simulink model "magnetorquer"  (R2021b)
settings: Solver=VariableStepAuto  StartTime=0.0  StopTime=10.0  RelTol=1e-3
libraries: matrix_library x2
settings Model: Creator=jorgemarrero  LastModifiedBy=jorgemarrero

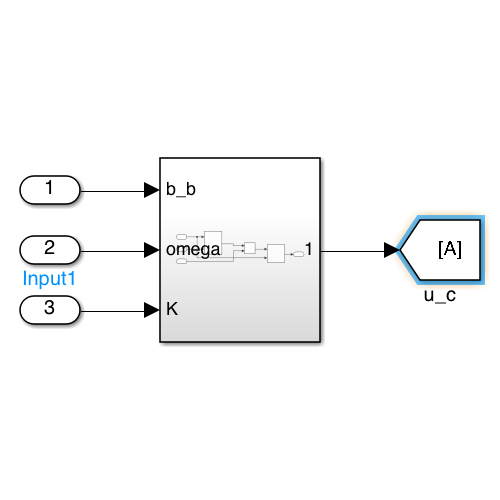
[thumbnail: Simulink's stored preview of the top-level diagram]
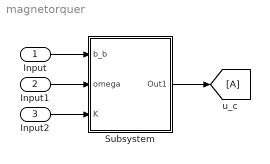
== system magnetorquer ==
  Input : Inport
  Input1 : Inport  Port=2
  Input2 : Inport  Port=3
  Subsystem : Subsystem
  wires:
  Input/1 -> Subsystem/1(b_b)
  Input1/1 -> Subsystem/2(omega)
  Subsystem/1(Out1) -> [A]
  Input2/1 -> Subsystem/3(K)

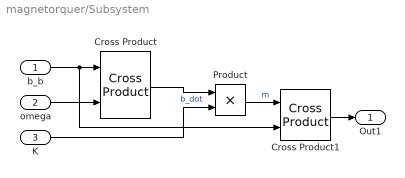
== system magnetorquer/Subsystem ==
  b_b : Inport
  omega : Inport  Port=2
  K : Inport  Port=3
  Cross Product : matrix_library/Cross Product
      settings: SourceProductBaseCode=SL
  Cross Product1 : matrix_library/Cross Product
      settings: SourceProductBaseCode=SL
  Product : Product
  Out1 : Outport
  wires:
  b_b/1 -> Cross Product1/2, Cross Product/1
  omega/1 -> Cross Product/2
  Cross Product/1 -> Product/1  "b_dot"
  K/1 -> Product/2
  Product/1 -> Cross Product1/1  "m"
  Cross Product1/1 -> Out1/1
